simulink model "sim_instalacja_podlogowa_modele_bojler"  (R2021b)
settings: Solver=VariableStepAuto  StartTime=0.0  StopTime=10.0  MaxStep=5  RelTol=1e-3
undefined symbols (not defined in the file): dRz_b, k, skok_czas2, T0_klasyczna, T_klasyczna
settings Model: Creator=adams  LastModifiedBy=adams

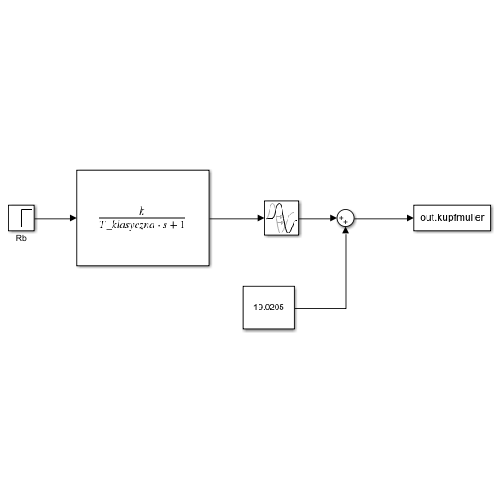
[thumbnail: Simulink's stored preview of the top-level diagram]
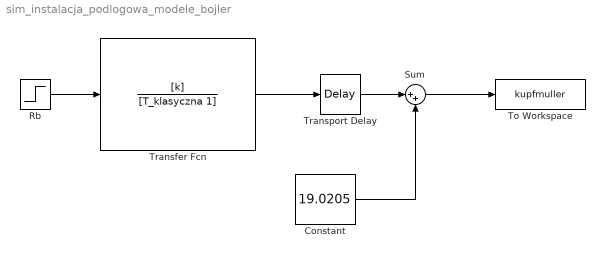
== system sim_instalacja_podlogowa_modele_bojler ==
  Constant : Constant  Value=19.0205
  Rb : Step  Time=skok_czas2  After=dRz_b  SampleTime=0
  Sum : Sum  Inputs=|++
  To Workspace : ToWorkspace  VariableName=kupfmuller  SampleTime=-1
  Transfer Fcn : TransferFcn  Numerator=[k]  Denominator=[T_klasyczna 1]
  Transport Delay : TransportDelay  DelayTime=T0_klasyczna  BufferSize=32768
  wires:
  Transfer Fcn/1 -> Transport Delay/1
  Constant/1 -> Sum/2
  Rb/1 -> Transfer Fcn/1
  Transport Delay/1 -> Sum/1
  Sum/1 -> To Workspace/1
